simulink library "multiTether_cl"  (R2018b)
settings: Solver=VariableStepAuto  StartTime=0.0  StopTime=10.0  RelTol=1e-3
undefined symbols (not defined in the file or in its folder): tether
libraries: singleTetherNGreater2_cl x1
settings Model: Creator=mcobb  LastModifiedBy=asiddiq2

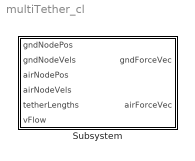
== system multiTether_cl ==
  Subsystem : Subsystem

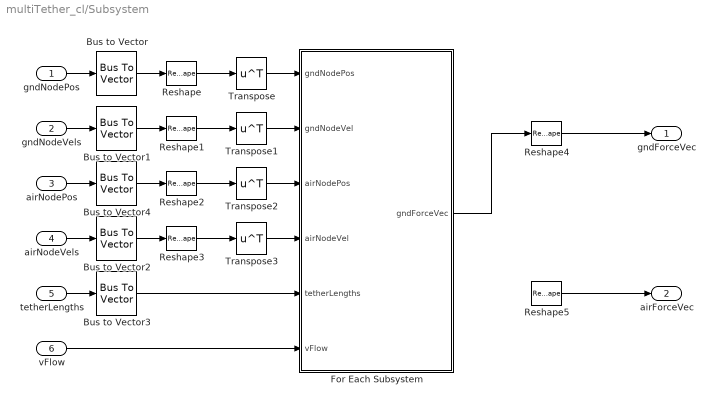
== system multiTether_cl/Subsystem ==
  gndNodePos : Inport
  gndNodeVels : Inport  Port=2
  airNodePos : Inport  Port=3
  airNodeVels : Inport  Port=4
  tetherLengths : Inport  Port=5
  vFlow : Inport  Port=6
  Bus to Vector{,1..4} (5 alike) : BusToVector
  For Each Subsystem : Subsystem  TreatAsAtomicUnit=on
  Reshape{,1..5} (6 alike) : Reshape  OutputDimensionality=Customize  OutputDimensions=[3,3]
  Transpose{,1..3} (4 alike) : Math  Operator=transpose  SaturateOnIntegerOverflow=on
  gndForceVec : Outport
  airForceVec : Outport  Port=2
  wires:
  gndNodePos/1 -> Bus to Vector/1
  tetherLengths/1 -> Bus to Vector3/1
  airNodeVels/1 -> Bus to Vector2/1
  airNodePos/1 -> Bus to Vector4/1
  gndNodeVels/1 -> Bus to Vector1/1
  For Each Subsystem/1(gndForceVec) -> Reshape4/1
  ? -> Reshape5/1
  Bus to Vector/1 -> Reshape/1
  Bus to Vector1/1 -> Reshape1/1
  Bus to Vector2/1 -> Reshape3/1
  Bus to Vector4/1 -> Reshape2/1
  Reshape/1 -> Transpose/1
  Reshape1/1 -> Transpose1/1
  Reshape2/1 -> Transpose2/1
  Reshape3/1 -> Transpose3/1
  Transpose/1 -> For Each Subsystem/1(gndNodePos)
  Transpose1/1 -> For Each Subsystem/2(gndNodeVel)
  Transpose2/1 -> For Each Subsystem/3(airNodePos)
  Transpose3/1 -> For Each Subsystem/4(airNodeVel)
  Bus to Vector3/1 -> For Each Subsystem/5(tetherLengths)
  vFlow/1 -> For Each Subsystem/6(vFlow)
  Reshape4/1 -> gndForceVec/1
  Reshape5/1 -> airForceVec/1

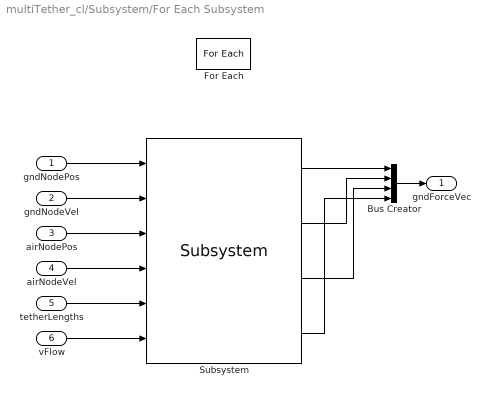
== system multiTether_cl/Subsystem/For Each Subsystem ==
  gndNodePos : Inport  Partition=on  PartitionDimension=1  PartitionWidth=1  PartitionOffset=0
  gndNodeVel : Inport  Port=2  Partition=on  PartitionDimension=1  PartitionWidth=1  PartitionOffset=0
  airNodePos : Inport  Port=3  Partition=on  PartitionDimension=1  PartitionWidth=1  PartitionOffset=0
  airNodeVel : Inport  Port=4  Partition=on  PartitionDimension=1  PartitionWidth=1  PartitionOffset=0
  tetherLengths : Inport  Port=5  Partition=on  PartitionDimension=1  PartitionWidth=1  PartitionOffset=0
  vFlow : Inport  Port=6
  Bus Creator : BusCreator  Inputs=4
  For Each : ForEach  DisableCoverage=on  IndexMode=One-based
  Subsystem : singleTetherNGreater2_cl/Subsystem  N=tether.N  dia_t=tether.diameter  E=tether.youngsMod  rho_tether=tether.density  Cd=tether.CD_Cyliner  zeta=tether.damping_ratio  rho=tether.fluidDensity  g=tether.gravity  mass=tether.vehicleMass  ini_Rn_o=tether.initAirPos  ini_R1_o=tether.initGndPos
  gndForceVec : Outport  ConcatenationDimension=1
  wires:
  gndNodePos/1 -> Subsystem/1
  gndNodeVel/1 -> Subsystem/2
  airNodeVel/1 -> Subsystem/4
  airNodePos/1 -> Subsystem/3
  tetherLengths/1 -> Subsystem/5
  vFlow/1 -> Subsystem/6
  Subsystem/1 -> Bus Creator/1
  Subsystem/2 -> Bus Creator/2
  Subsystem/3 -> Bus Creator/3
  Subsystem/4 -> Bus Creator/4
  Bus Creator/1 -> gndForceVec/1
